simulink model "single_fre_transmit"  (R2022a)
settings: Solver=FixedStepDiscrete  StartTime=0.0  StopTime=1  FixedStep=0.01  RelTol=1e-3
model workspace (MAT data in the model file):
  amplitude = 1
  fc = 1000
settings Model: Creator=luoch  LastModifiedBy=luoch
settings DataIOCC: SaveOutput=off  SignalLogging=off
settings ModelReferenceCC: EnableRefExpFcnMdlSchedulingChecks=off
settings RTWCC: Description=Generic Real-Time Target  GPUComputeCapability=5.0
settings ConfigComp: CovBoundaryAbsTol=1.0e-5

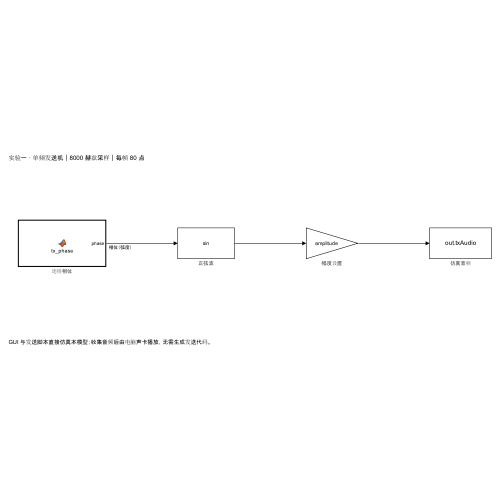
[thumbnail: Simulink's stored preview of the top-level diagram]
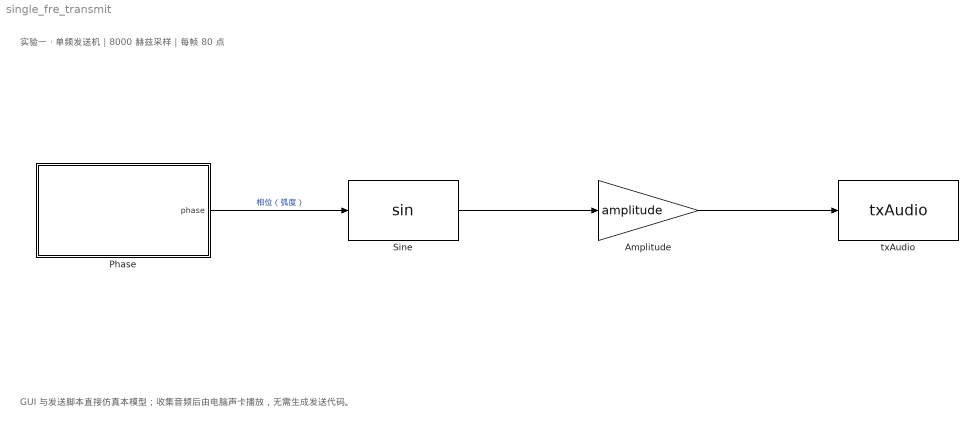
== system single_fre_transmit ==
  note: 实验一 · 单频发送机｜8000 赫兹采样｜每帧 80 点
  note: GUI 与发送脚本直接仿真本模型；收集音频后由电脑声卡播放，无需生成发送代码。
  Amplitude : Gain  Gain=amplitude
      settings: AttributesFormatString=幅度设置
  Phase : MATLAB Function  TreatAsAtomicUnit=on
      settings: AttributesFormatString=连续相位
  Sine : Trigonometry
      settings: AttributesFormatString=正弦波
  txAudio : ToWorkspace  VariableName=txAudio  SampleTime=-1
      settings: AttributesFormatString=仿真音频
  wires:
  Phase/1(phase) -> Sine/1  "相位（弧度）"
  Sine/1 -> Amplitude/1
  Amplitude/1 -> txAudio/1

== matlab function single_fre_transmit/Phase ==
  settings: updateMethod=DISCRETE  sampleTime=0.01
  data: phase output; fc parameter
function phase=tx_phase(fc)
%#codegen
% 每次推进 80 个采样，相位沿整段波形连续。
persistent sample
if isempty(sample),sample=0;end
phase=2*pi*fc*(sample+(0:79)')/8000;sample=sample+80;
end
